simulink model "VU_lineFollow"  (Simulink 10.0)
settings: Solver=FixedStepDiscrete  StartTime=0.0  StopTime=inf  FixedStep=0.1  RelTol=1e-3  EnableMultiTasking=on
libraries: lego_nxt_lib x3
settings Model: Creator=jpeytonj  LastModifiedBy=bhisma
settings DataIOCC: LimitDataPoints=on  SignalLoggingSaveFormat=ModelDataLogs
settings OptimizationCC: ExpressionDepthLimit=2147483647
settings DebuggingCC: SolverPrmCheckMsg=warning  FcnCallInpInsideContextMsg=warning  StateNameClashWarn=warning
settings SFSimCC: SimParseCustomCode=off
settings RTWCC: Description=Lego NXT Real-Time Target  SystemTargetFile=lrt.tlc  GenCodeOnly=on  TemplateMakefile=lrt_ecrobot.tmf
settings STFCustomTargetCC: ModelReferenceCompliant=off  GeneratePreprocessorConditionals=Disable all  MatFileLogging=on  CPPClassGenCompliant=on  SystemTargetFile=lrt.tlc
settings GRTTargetCC: ModelReferenceCompliant=off  ParMdlRefBuildCompliant=off  CompOptLevelCompliant=off  ConcurrentExecutionCompliant=off  GeneratePreprocessorConditionals=Disable all  UseToolchainInfoCompliant=off  ExtModeMexFile=noextcomm
settings CustomProperty: DataType=RTWOptions_EnumType_C__RTtools_VU-LRT_lrt_1codeGenType  Value=Integer-only
settings EnumStrPairs: String=Integer-only
settings ConfigComp: CovExternalEMLEnable=off

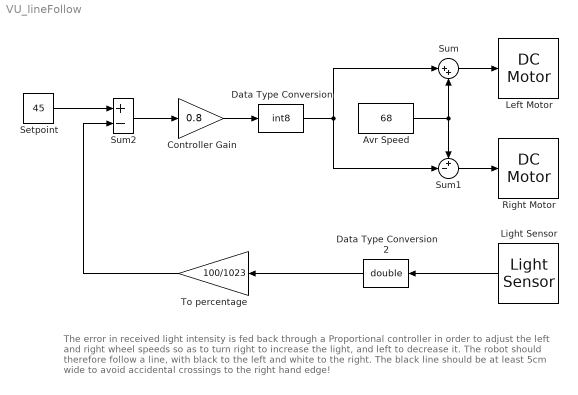
== system VU_lineFollow ==
  note: The error in received light intensity is fed back through a Proportional controller in order to adjust
      | the left and right wheel speeds so as to turn right to increase the light, and left to decrease it.
      | The robot should therefore follow a line, with black to the left and white to the right.
      | The black line should be at least 5cm wide to avoid accidental crossings to the right hand edge!
  Avr Speed : Constant  Value=68  OutDataTypeStr=int8
  Controller Gain : Gain  Gain=0.8
  Data Type Conversion : DataTypeConversion  OutDataTypeStr=int8  SaturateOnIntegerOverflow=on
  Data Type Conversion2 : DataTypeConversion  OutDataTypeStr=double  SaturateOnIntegerOverflow=on
  Left Motor : lego_nxt_lib/DC Motor  port=Port C  brake=Coast
  Light Sensor : lego_nxt_lib/Light Sensor  port=Port 3  st=-1
  Right Motor : lego_nxt_lib/DC Motor  port=Port B  brake=Coast
  Setpoint : Constant  Value=45
  Sum : Sum  Inputs=|++
  Sum1 : Sum  Inputs=+-|
  Sum2 : Sum  Inputs=+-
  To percentage : Gain  Gain=100/1023
  wires:
  Controller Gain/1 -> Data Type Conversion/1
  Setpoint/1 -> Sum2/1
  Data Type Conversion/1 -> Sum/1, Sum1/2
  Avr Speed/1 -> Sum/2, Sum1/1
  Sum/1 -> Left Motor/1
  Sum1/1 -> Right Motor/1
  Light Sensor/1 -> Data Type Conversion2/1
  Data Type Conversion2/1 -> To percentage/1
  Sum2/1 -> Controller Gain/1
  To percentage/1 -> Sum2/2
